simulink model "example"  (Simulink 7.0)
settings: Solver=ode4  StartTime=0.0  StopTime=100  FixedStep=0.01  RelTol=1e-3
values from neighbouring files (symbols this model uses):
  TID = min('TI' == AFT(1:2))    [PAS_callback.m]    (also in PSTID_callback.m = [block '/TID'])
libraries: simulink x280
(part 2 of 15)

== system example/<system name>/<Requirement name>/<Preconditions name>4 ==
  InOut Bus : Inport  OutDataType=sfix(16)  OutScaling=2^0
  <Reference name> : Constant  OutDataType=sfix(16)  OutScaling=2^0
  Bus Selector : BusSelector  OutputSignals=signal1
  Feature extraction : Subsystem  TreatAsAtomicUnit=on  mask{Param=0}
      mask prompts: Param "Mask Parameter 1:"
  PS : Subsystem  mask(Feature layer: preconditions synchronization){NoTI=0, NoTDD=0, NoTID=1, TIdel=[0], TDDdel=[0]}
      mask prompts: NoTI "Time-independent features identifiable with or without a delay (TI)"; NoTDD "Triggered features identifiable with determinate delay or without a delay (TDD)"; NoTID "Triggered features identifiable with indeterminate delay (TID)"; TIdel "Time-independent features delays (in time steps). E.g. [0 1 0] for 3 features"; TDDdel "Triggered features delays (in time steps). E.g. [0 0] for 2 features"
      mask help: Use this block for synchronizing the precondition features. For changing the block inputs, use the parameters below. The output must be used for assertions activation.
      mask init:
      | PS_init(gcb);
      mask StyleString: popup(0|1|2|3|4|5|6|7|8|9),popup(0|1|2|3|4|5|6|7|8|9),popup(0|1|2|3|4|5|6|7|8|9),edit,edit
      mask CallbackString:
      | PSTI_callback(gcb);|PSTDD_callback(gcb);|PSTID_callback(gcb);|NoTI = str2double(get_param(gcb,'NoTI'));
      | TIdel = str2num(get_param(gcb,'TIdel'));
      | if NoTI ~= length(TIdel) && NoTI ~= 0
      |     error(['The number of delays entered (' num2str(length(TIdel)) ') does not correspond to the above specified number of time-independent features (' num2str(NoTI) ').']);
      | end|NoTDD = str2double(get_param(gcb,'NoTDD'));
      | TDDdel = str2num(get_param(gcb,'TDDdel'));
      | if NoTDD ~= length(TDDdel) && NoTDD ~= 0
      |     error(['The number of delays entered (' num2str(length(TDDdel)) ') does not correspond to the above specified number of triggered features with constant delay (' num2str(NoTDD) ').']);
      | end
  Signal comparison : Subsystem  TreatAsAtomicUnit=on  mask{Param=0}
      mask prompts: Param "Mask Parameter 1:"
  Activate : Outport  OutDataType=sfix(16)  OutScaling=2^0
  wires:
  InOut Bus/1 -> Bus Selector/1
  PS/1(Precond) -> Activate/1
  Signal comparison/1(A) -> PS/3(A TID1)
  <Reference name>/1 -> Signal comparison/2(Ref)
  Feature extraction/3(A) -> Signal comparison/1(Sig)
  Feature extraction/2(T) -> PS/2(T TID1)
  Feature extraction/1(R) -> PS/1(R TID1)
  Bus Selector/1 -> Feature extraction/1(Sig)  "<signal1>"

== system example/<system name>/<Requirement name>/<Preconditions name>5 ==
  InOut Bus : Inport  OutDataType=sfix(16)  OutScaling=2^0
  <Reference name> : Constant  OutDataType=sfix(16)  OutScaling=2^0
  Bus Selector : BusSelector  OutputSignals=signal1
  Feature extraction : Subsystem  TreatAsAtomicUnit=on  mask{Param=0}
      mask prompts: Param "Mask Parameter 1:"
  PS : Subsystem  mask(Feature layer: preconditions synchronization){NoTI=0, NoTDD=0, NoTID=1, TIdel=[0], TDDdel=[0]}
      mask prompts: NoTI "Time-independent features identifiable with or without a delay (TI)"; NoTDD "Triggered features identifiable with determinate delay or without a delay (TDD)"; NoTID "Triggered features identifiable with indeterminate delay (TID)"; TIdel "Time-independent features delays (in time steps). E.g. [0 1 0] for 3 features"; TDDdel "Triggered features delays (in time steps). E.g. [0 0] for 2 features"
      mask help: Use this block for synchronizing the precondition features. For changing the block inputs, use the parameters below. The output must be used for assertions activation.
      mask init:
      | PS_init(gcb);
      mask StyleString: popup(0|1|2|3|4|5|6|7|8|9),popup(0|1|2|3|4|5|6|7|8|9),popup(0|1|2|3|4|5|6|7|8|9),edit,edit
      mask CallbackString:
      | PSTI_callback(gcb);|PSTDD_callback(gcb);|PSTID_callback(gcb);|NoTI = str2double(get_param(gcb,'NoTI'));
      | TIdel = str2num(get_param(gcb,'TIdel'));
      | if NoTI ~= length(TIdel) && NoTI ~= 0
      |     error(['The number of delays entered (' num2str(length(TIdel)) ') does not correspond to the above specified number of time-independent features (' num2str(NoTI) ').']);
      | end|NoTDD = str2double(get_param(gcb,'NoTDD'));
      | TDDdel = str2num(get_param(gcb,'TDDdel'));
      | if NoTDD ~= length(TDDdel) && NoTDD ~= 0
      |     error(['The number of delays entered (' num2str(length(TDDdel)) ') does not correspond to the above specified number of triggered features with constant delay (' num2str(NoTDD) ').']);
      | end
  Signal comparison : Subsystem  TreatAsAtomicUnit=on  mask{Param=0}
      mask prompts: Param "Mask Parameter 1:"
  Activate : Outport  OutDataType=sfix(16)  OutScaling=2^0
  wires:
  InOut Bus/1 -> Bus Selector/1
  PS/1(Precond) -> Activate/1
  Signal comparison/1(A) -> PS/3(A TID1)
  <Reference name>/1 -> Signal comparison/2(Ref)
  Feature extraction/3(A) -> Signal comparison/1(Sig)
  Feature extraction/2(T) -> PS/2(T TID1)
  Feature extraction/1(R) -> PS/1(R TID1)
  Bus Selector/1 -> Feature extraction/1(Sig)  "<signal1>"

== system example/<system name>/<Requirement name>/<Preconditions name>6 ==
  InOut Bus : Inport  OutDataType=sfix(16)  OutScaling=2^0
  <Reference name> : Constant  OutDataType=sfix(16)  OutScaling=2^0
  Bus Selector : BusSelector  OutputSignals=signal1
  Feature extraction : Subsystem  TreatAsAtomicUnit=on  mask{Param=0}
      mask prompts: Param "Mask Parameter 1:"
  PS : Subsystem  mask(Feature layer: preconditions synchronization){NoTI=0, NoTDD=0, NoTID=1, TIdel=[0], TDDdel=[0]}
      mask prompts: NoTI "Time-independent features identifiable with or without a delay (TI)"; NoTDD "Triggered features identifiable with determinate delay or without a delay (TDD)"; NoTID "Triggered features identifiable with indeterminate delay (TID)"; TIdel "Time-independent features delays (in time steps). E.g. [0 1 0] for 3 features"; TDDdel "Triggered features delays (in time steps). E.g. [0 0] for 2 features"
      mask help: Use this block for synchronizing the precondition features. For changing the block inputs, use the parameters below. The output must be used for assertions activation.
      mask init:
      | PS_init(gcb);
      mask StyleString: popup(0|1|2|3|4|5|6|7|8|9),popup(0|1|2|3|4|5|6|7|8|9),popup(0|1|2|3|4|5|6|7|8|9),edit,edit
      mask CallbackString:
      | PSTI_callback(gcb);|PSTDD_callback(gcb);|PSTID_callback(gcb);|NoTI = str2double(get_param(gcb,'NoTI'));
      | TIdel = str2num(get_param(gcb,'TIdel'));
      | if NoTI ~= length(TIdel) && NoTI ~= 0
      |     error(['The number of delays entered (' num2str(length(TIdel)) ') does not correspond to the above specified number of time-independent features (' num2str(NoTI) ').']);
      | end|NoTDD = str2double(get_param(gcb,'NoTDD'));
      | TDDdel = str2num(get_param(gcb,'TDDdel'));
      | if NoTDD ~= length(TDDdel) && NoTDD ~= 0
      |     error(['The number of delays entered (' num2str(length(TDDdel)) ') does not correspond to the above specified number of triggered features with constant delay (' num2str(NoTDD) ').']);
      | end
  Signal comparison : Subsystem  TreatAsAtomicUnit=on  mask{Param=0}
      mask prompts: Param "Mask Parameter 1:"
  Activate : Outport  OutDataType=sfix(16)  OutScaling=2^0
  wires:
  InOut Bus/1 -> Bus Selector/1
  PS/1(Precond) -> Activate/1
  Signal comparison/1(A) -> PS/3(A TID1)
  <Reference name>/1 -> Signal comparison/2(Ref)
  Feature extraction/3(A) -> Signal comparison/1(Sig)
  Feature extraction/2(T) -> PS/2(T TID1)
  Feature extraction/1(R) -> PS/1(R TID1)
  Bus Selector/1 -> Feature extraction/1(Sig)  "<signal1>"

== system example/<system name>/<Requirement name>2/<Assertions name> ==
  Precond : Inport  OutDataType=sfix(16)  OutScaling=2^0
  InOut Bus : Inport  Port=2  OutDataType=sfix(16)  OutScaling=2^0
  <Reference name> : Constant  OutDataType=sfix(16)  OutScaling=2^0
  Bus Creator : BusCreator  Inputs=1
  Bus Selector : BusSelector  OutputSignals=signal1
  Feature extraction : Subsystem  TreatAsAtomicUnit=on  mask{Param=0}
      mask prompts: Param "Mask Parameter 1:"
  PAS : Subsystem  mask{AFT=TID, AFD=600}
      mask prompts: AFT "Assertion feature type:"; AFD "Assertion feature delay (in time steps)"
      mask init:
      | PAS_init(gcb);
      mask StyleString: popup(TI|TDD|TID),edit
      mask CallbackString: PAS_callback(gcb);|
  Signal comparison : Subsystem  TreatAsAtomicUnit=on  mask{Param=0}
      mask prompts: Param "Mask Parameter 1:"
  VF info : Outport  OutDataType=sfix(16)  OutScaling=2^0
  wires:
  Bus Creator/1 -> VF info/1
  InOut Bus/1 -> Bus Selector/1
  Precond/1 -> PAS/1(Precond)
  PAS/1(VF Info) -> Bus Creator/1
  <Reference name>/1 -> Signal comparison/2(Ref)
  Feature extraction/3(A) -> Signal comparison/1(Sig)
  Feature extraction/2(T) -> PAS/3(T)
  Feature extraction/1(R) -> PAS/2(R)
  Bus Selector/1 -> Feature extraction/1(Sig)  "<signal1>"
  Signal comparison/1(V) -> PAS/4(V)

== system example/<system name>/<Requirement name>2/<Preconditions name> ==
  InOut Bus : Inport  OutDataType=sfix(16)  OutScaling=2^0
  <Reference name> : Constant  OutDataType=sfix(16)  OutScaling=2^0
  Bus Selector : BusSelector  OutputSignals=signal1
  Feature extraction : Subsystem  TreatAsAtomicUnit=on  mask{Param=0}
      mask prompts: Param "Mask Parameter 1:"
  PS : Subsystem  mask(Feature layer: preconditions synchronization){NoTI=0, NoTDD=0, NoTID=1, TIdel=[0], TDDdel=[0]}
      mask prompts: NoTI "Time-independent features identifiable with or without a delay (TI)"; NoTDD "Triggered features identifiable with determinate delay or without a delay (TDD)"; NoTID "Triggered features identifiable with indeterminate delay (TID)"; TIdel "Time-independent features delays (in time steps). E.g. [0 1 0] for 3 features"; TDDdel "Triggered features delays (in time steps). E.g. [0 0] for 2 features"
      mask help: Use this block for synchronizing the precondition features. For changing the block inputs, use the parameters below. The output must be used for assertions activation.
      mask init:
      | PS_init(gcb);
      mask StyleString: popup(0|1|2|3|4|5|6|7|8|9),popup(0|1|2|3|4|5|6|7|8|9),popup(0|1|2|3|4|5|6|7|8|9),edit,edit
      mask CallbackString:
      | PSTI_callback(gcb);|PSTDD_callback(gcb);|PSTID_callback(gcb);|NoTI = str2double(get_param(gcb,'NoTI'));
      | TIdel = str2num(get_param(gcb,'TIdel'));
      | if NoTI ~= length(TIdel) && NoTI ~= 0
      |     error(['The number of delays entered (' num2str(length(TIdel)) ') does not correspond to the above specified number of time-independent features (' num2str(NoTI) ').']);
      | end|NoTDD = str2double(get_param(gcb,'NoTDD'));
      | TDDdel = str2num(get_param(gcb,'TDDdel'));
      | if NoTDD ~= length(TDDdel) && NoTDD ~= 0
      |     error(['The number of delays entered (' num2str(length(TDDdel)) ') does not correspond to the above specified number of triggered features with constant delay (' num2str(NoTDD) ').']);
      | end
  Signal comparison : Subsystem  TreatAsAtomicUnit=on  mask{Param=0}
      mask prompts: Param "Mask Parameter 1:"
  Activate : Outport  OutDataType=sfix(16)  OutScaling=2^0
  wires:
  InOut Bus/1 -> Bus Selector/1
  PS/1(Precond) -> Activate/1
  Signal comparison/1(A) -> PS/3(A TID1)
  <Reference name>/1 -> Signal comparison/2(Ref)
  Feature extraction/3(A) -> Signal comparison/1(Sig)
  Feature extraction/2(T) -> PS/2(T TID1)
  Feature extraction/1(R) -> PS/1(R TID1)
  Bus Selector/1 -> Feature extraction/1(Sig)  "<signal1>"

== system example/<system name>/<Requirement name>3/<Assertions name> ==
  Precond : Inport  OutDataType=sfix(16)  OutScaling=2^0
  InOut Bus : Inport  Port=2  OutDataType=sfix(16)  OutScaling=2^0
  <Reference name> : Constant  OutDataType=sfix(16)  OutScaling=2^0
  Bus Creator : BusCreator  Inputs=1
  Bus Selector : BusSelector  OutputSignals=signal1
  Feature extraction : Subsystem  TreatAsAtomicUnit=on  mask{Param=0}
      mask prompts: Param "Mask Parameter 1:"
  PAS : Subsystem  mask{AFT=TID, AFD=600}
      mask prompts: AFT "Assertion feature type:"; AFD "Assertion feature delay (in time steps)"
      mask init:
      | PAS_init(gcb);
      mask StyleString: popup(TI|TDD|TID),edit
      mask CallbackString: PAS_callback(gcb);|
  Signal comparison : Subsystem  TreatAsAtomicUnit=on  mask{Param=0}
      mask prompts: Param "Mask Parameter 1:"
  VF info : Outport  OutDataType=sfix(16)  OutScaling=2^0
  wires:
  Bus Creator/1 -> VF info/1
  InOut Bus/1 -> Bus Selector/1
  Precond/1 -> PAS/1(Precond)
  PAS/1(VF Info) -> Bus Creator/1
  <Reference name>/1 -> Signal comparison/2(Ref)
  Feature extraction/3(A) -> Signal comparison/1(Sig)
  Feature extraction/2(T) -> PAS/3(T)
  Feature extraction/1(R) -> PAS/2(R)
  Bus Selector/1 -> Feature extraction/1(Sig)  "<signal1>"
  Signal comparison/1(V) -> PAS/4(V)

== system example/<system name>/<Requirement name>3/<Preconditions name> ==
  InOut Bus : Inport  OutDataType=sfix(16)  OutScaling=2^0
  <Reference name> : Constant  OutDataType=sfix(16)  OutScaling=2^0
  Bus Selector : BusSelector  OutputSignals=signal1
  Feature extraction : Subsystem  TreatAsAtomicUnit=on  mask{Param=0}
      mask prompts: Param "Mask Parameter 1:"
  PS : Subsystem  mask(Feature layer: preconditions synchronization){NoTI=0, NoTDD=0, NoTID=1, TIdel=[0], TDDdel=[0]}
      mask prompts: NoTI "Time-independent features identifiable with or without a delay (TI)"; NoTDD "Triggered features identifiable with determinate delay or without a delay (TDD)"; NoTID "Triggered features identifiable with indeterminate delay (TID)"; TIdel "Time-independent features delays (in time steps). E.g. [0 1 0] for 3 features"; TDDdel "Triggered features delays (in time steps). E.g. [0 0] for 2 features"
      mask help: Use this block for synchronizing the precondition features. For changing the block inputs, use the parameters below. The output must be used for assertions activation.
      mask init:
      | PS_init(gcb);
      mask StyleString: popup(0|1|2|3|4|5|6|7|8|9),popup(0|1|2|3|4|5|6|7|8|9),popup(0|1|2|3|4|5|6|7|8|9),edit,edit
      mask CallbackString:
      | PSTI_callback(gcb);|PSTDD_callback(gcb);|PSTID_callback(gcb);|NoTI = str2double(get_param(gcb,'NoTI'));
      | TIdel = str2num(get_param(gcb,'TIdel'));
      | if NoTI ~= length(TIdel) && NoTI ~= 0
      |     error(['The number of delays entered (' num2str(length(TIdel)) ') does not correspond to the above specified number of time-independent features (' num2str(NoTI) ').']);
      | end|NoTDD = str2double(get_param(gcb,'NoTDD'));
      | TDDdel = str2num(get_param(gcb,'TDDdel'));
      | if NoTDD ~= length(TDDdel) && NoTDD ~= 0
      |     error(['The number of delays entered (' num2str(length(TDDdel)) ') does not correspond to the above specified number of triggered features with constant delay (' num2str(NoTDD) ').']);
      | end
  Signal comparison : Subsystem  TreatAsAtomicUnit=on  mask{Param=0}
      mask prompts: Param "Mask Parameter 1:"
  Activate : Outport  OutDataType=sfix(16)  OutScaling=2^0
  wires:
  InOut Bus/1 -> Bus Selector/1
  PS/1(Precond) -> Activate/1
  Signal comparison/1(A) -> PS/3(A TID1)
  <Reference name>/1 -> Signal comparison/2(Ref)
  Feature extraction/3(A) -> Signal comparison/1(Sig)
  Feature extraction/2(T) -> PS/2(T TID1)
  Feature extraction/1(R) -> PS/1(R TID1)
  Bus Selector/1 -> Feature extraction/1(Sig)  "<signal1>"

== system example/<system name>/<Requirement name>4/<Assertions name> ==
  Precond : Inport  OutDataType=sfix(16)  OutScaling=2^0
  InOut Bus : Inport  Port=2  OutDataType=sfix(16)  OutScaling=2^0
  <Reference name> : Constant  OutDataType=sfix(16)  OutScaling=2^0
  Bus Creator : BusCreator  Inputs=1
  Bus Selector : BusSelector  OutputSignals=signal1
  Feature extraction : Subsystem  TreatAsAtomicUnit=on  mask{Param=0}
      mask prompts: Param "Mask Parameter 1:"
  PAS : Subsystem  mask{AFT=TID, AFD=600}
      mask prompts: AFT "Assertion feature type:"; AFD "Assertion feature delay (in time steps)"
      mask init:
      | PAS_init(gcb);
      mask StyleString: popup(TI|TDD|TID),edit
      mask CallbackString: PAS_callback(gcb);|
  Signal comparison : Subsystem  TreatAsAtomicUnit=on  mask{Param=0}
      mask prompts: Param "Mask Parameter 1:"
  VF info : Outport  OutDataType=sfix(16)  OutScaling=2^0
  wires:
  Bus Creator/1 -> VF info/1
  InOut Bus/1 -> Bus Selector/1
  Precond/1 -> PAS/1(Precond)
  PAS/1(VF Info) -> Bus Creator/1
  <Reference name>/1 -> Signal comparison/2(Ref)
  Feature extraction/3(A) -> Signal comparison/1(Sig)
  Feature extraction/2(T) -> PAS/3(T)
  Feature extraction/1(R) -> PAS/2(R)
  Bus Selector/1 -> Feature extraction/1(Sig)  "<signal1>"
  Signal comparison/1(V) -> PAS/4(V)

== system example/<system name>/<Requirement name>4/<Preconditions name> ==
  InOut Bus : Inport  OutDataType=sfix(16)  OutScaling=2^0
  <Reference name> : Constant  OutDataType=sfix(16)  OutScaling=2^0
  Bus Selector : BusSelector  OutputSignals=signal1
  Feature extraction : Subsystem  TreatAsAtomicUnit=on  mask{Param=0}
      mask prompts: Param "Mask Parameter 1:"
  PS : Subsystem  mask(Feature layer: preconditions synchronization){NoTI=0, NoTDD=0, NoTID=1, TIdel=[0], TDDdel=[0]}
      mask prompts: NoTI "Time-independent features identifiable with or without a delay (TI)"; NoTDD "Triggered features identifiable with determinate delay or without a delay (TDD)"; NoTID "Triggered features identifiable with indeterminate delay (TID)"; TIdel "Time-independent features delays (in time steps). E.g. [0 1 0] for 3 features"; TDDdel "Triggered features delays (in time steps). E.g. [0 0] for 2 features"
      mask help: Use this block for synchronizing the precondition features. For changing the block inputs, use the parameters below. The output must be used for assertions activation.
      mask init:
      | PS_init(gcb);
      mask StyleString: popup(0|1|2|3|4|5|6|7|8|9),popup(0|1|2|3|4|5|6|7|8|9),popup(0|1|2|3|4|5|6|7|8|9),edit,edit
      mask CallbackString:
      | PSTI_callback(gcb);|PSTDD_callback(gcb);|PSTID_callback(gcb);|NoTI = str2double(get_param(gcb,'NoTI'));
      | TIdel = str2num(get_param(gcb,'TIdel'));
      | if NoTI ~= length(TIdel) && NoTI ~= 0
      |     error(['The number of delays entered (' num2str(length(TIdel)) ') does not correspond to the above specified number of time-independent features (' num2str(NoTI) ').']);
      | end|NoTDD = str2double(get_param(gcb,'NoTDD'));
      | TDDdel = str2num(get_param(gcb,'TDDdel'));
      | if NoTDD ~= length(TDDdel) && NoTDD ~= 0
      |     error(['The number of delays entered (' num2str(length(TDDdel)) ') does not correspond to the above specified number of triggered features with constant delay (' num2str(NoTDD) ').']);
      | end
  Signal comparison : Subsystem  TreatAsAtomicUnit=on  mask{Param=0}
      mask prompts: Param "Mask Parameter 1:"
  Activate : Outport  OutDataType=sfix(16)  OutScaling=2^0
  wires:
  InOut Bus/1 -> Bus Selector/1
  PS/1(Precond) -> Activate/1
  Signal comparison/1(A) -> PS/3(A TID1)
  <Reference name>/1 -> Signal comparison/2(Ref)
  Feature extraction/3(A) -> Signal comparison/1(Sig)
  Feature extraction/2(T) -> PS/2(T TID1)
  Feature extraction/1(R) -> PS/1(R TID1)
  Bus Selector/1 -> Feature extraction/1(Sig)  "<signal1>"

== system example/<system name>/<Requirement name>5/<Assertions name> ==
  Precond : Inport  OutDataType=sfix(16)  OutScaling=2^0
  InOut Bus : Inport  Port=2  OutDataType=sfix(16)  OutScaling=2^0
  <Reference name> : Constant  OutDataType=sfix(16)  OutScaling=2^0
  Bus Creator : BusCreator  Inputs=1
  Bus Selector : BusSelector  OutputSignals=signal1
  Feature extraction : Subsystem  TreatAsAtomicUnit=on  mask{Param=0}
      mask prompts: Param "Mask Parameter 1:"
  PAS : Subsystem  mask{AFT=TID, AFD=600}
      mask prompts: AFT "Assertion feature type:"; AFD "Assertion feature delay (in time steps)"
      mask init:
      | PAS_init(gcb);
      mask StyleString: popup(TI|TDD|TID),edit
      mask CallbackString: PAS_callback(gcb);|
  Signal comparison : Subsystem  TreatAsAtomicUnit=on  mask{Param=0}
      mask prompts: Param "Mask Parameter 1:"
  VF info : Outport  OutDataType=sfix(16)  OutScaling=2^0
  wires:
  Bus Creator/1 -> VF info/1
  InOut Bus/1 -> Bus Selector/1
  Precond/1 -> PAS/1(Precond)
  PAS/1(VF Info) -> Bus Creator/1
  <Reference name>/1 -> Signal comparison/2(Ref)
  Feature extraction/3(A) -> Signal comparison/1(Sig)
  Feature extraction/2(T) -> PAS/3(T)
  Feature extraction/1(R) -> PAS/2(R)
  Bus Selector/1 -> Feature extraction/1(Sig)  "<signal1>"
  Signal comparison/1(V) -> PAS/4(V)

== system example/<system name>/<Requirement name>5/<Preconditions name> ==
  InOut Bus : Inport  OutDataType=sfix(16)  OutScaling=2^0
  <Reference name> : Constant  OutDataType=sfix(16)  OutScaling=2^0
  Bus Selector : BusSelector  OutputSignals=signal1
  Feature extraction : Subsystem  TreatAsAtomicUnit=on  mask{Param=0}
      mask prompts: Param "Mask Parameter 1:"
  PS : Subsystem  mask(Feature layer: preconditions synchronization){NoTI=0, NoTDD=0, NoTID=1, TIdel=[0], TDDdel=[0]}
      mask prompts: NoTI "Time-independent features identifiable with or without a delay (TI)"; NoTDD "Triggered features identifiable with determinate delay or without a delay (TDD)"; NoTID "Triggered features identifiable with indeterminate delay (TID)"; TIdel "Time-independent features delays (in time steps). E.g. [0 1 0] for 3 features"; TDDdel "Triggered features delays (in time steps). E.g. [0 0] for 2 features"
      mask help: Use this block for synchronizing the precondition features. For changing the block inputs, use the parameters below. The output must be used for assertions activation.
      mask init:
      | PS_init(gcb);
      mask StyleString: popup(0|1|2|3|4|5|6|7|8|9),popup(0|1|2|3|4|5|6|7|8|9),popup(0|1|2|3|4|5|6|7|8|9),edit,edit
      mask CallbackString:
      | PSTI_callback(gcb);|PSTDD_callback(gcb);|PSTID_callback(gcb);|NoTI = str2double(get_param(gcb,'NoTI'));
      | TIdel = str2num(get_param(gcb,'TIdel'));
      | if NoTI ~= length(TIdel) && NoTI ~= 0
      |     error(['The number of delays entered (' num2str(length(TIdel)) ') does not correspond to the above specified number of time-independent features (' num2str(NoTI) ').']);
      | end|NoTDD = str2double(get_param(gcb,'NoTDD'));
      | TDDdel = str2num(get_param(gcb,'TDDdel'));
      | if NoTDD ~= length(TDDdel) && NoTDD ~= 0
      |     error(['The number of delays entered (' num2str(length(TDDdel)) ') does not correspond to the above specified number of triggered features with constant delay (' num2str(NoTDD) ').']);
      | end
  Signal comparison : Subsystem  TreatAsAtomicUnit=on  mask{Param=0}
      mask prompts: Param "Mask Parameter 1:"
  Activate : Outport  OutDataType=sfix(16)  OutScaling=2^0
  wires:
  InOut Bus/1 -> Bus Selector/1
  PS/1(Precond) -> Activate/1
  Signal comparison/1(A) -> PS/3(A TID1)
  <Reference name>/1 -> Signal comparison/2(Ref)
  Feature extraction/3(A) -> Signal comparison/1(Sig)
  Feature extraction/2(T) -> PS/2(T TID1)
  Feature extraction/1(R) -> PS/1(R TID1)
  Bus Selector/1 -> Feature extraction/1(Sig)  "<signal1>"

== system example/<Test data generator>/<Requirement name>/<Preconditions name>/<Check> ==
  Out Bus : Inport  OutDataType=sfix(16)  OutScaling=2^0
  <Reference name> : Constant  OutDataType=sfix(16)  OutScaling=2^0
  Bus Selector : BusSelector  OutputSignals=signal1
  Memory : Memory  X0=[1]
  Signal comparison : Subsystem  TreatAsAtomicUnit=on  mask{Param=0}
      mask prompts: Param "Mask Parameter 1:"
  A : Outport  OutDataType=sfix(16)  OutScaling=2^0
  wires:
  Out Bus/1 -> Bus Selector/1
  Signal comparison/1(A) -> A/1
  Memory/1 -> Signal comparison/1(Sig)
  <Reference name>/1 -> Signal comparison/2(Ref)
  Bus Selector/1 -> Memory/1  "<SUT output>"

== system example/<Test data generator>/<Requirement name>/<Preconditions name>/Feature generation ==
  <signal1> : Outport  OutDataType=sfix(16)  OutScaling=2^0

== system example/<Test data generator>/<Requirement name>/<Preconditions name>/Feature generation2 ==
  <signal1> : Outport  OutDataType=sfix(16)  OutScaling=2^0

== system example/<Test data generator>/<Requirement name>/<Preconditions name>/Feature generation3 ==
  <signal1> : Outport  OutDataType=sfix(16)  OutScaling=2^0

== system example/<Test data generator>/<Requirement name>/<Preconditions name>/Feature generation4 ==
  <signal1> : Outport  OutDataType=sfix(16)  OutScaling=2^0

== system example/<Test data generator>/<Requirement name>/<Preconditions name>/Feature generation5 ==
  <signal1> : Outport  OutDataType=sfix(16)  OutScaling=2^0

== system example/<Test data generator>/<Requirement name>/<Preconditions name>/Feature generation6 ==
  <signal1> : Outport  OutDataType=sfix(16)  OutScaling=2^0

== system example/<Test data generator>/<Requirement name>/<Preconditions name>/Feature generation7 ==
  <signal1> : Outport  OutDataType=sfix(16)  OutScaling=2^0

== system example/<Test data generator>/<Requirement name>/Initialisation & Stabilisation/<Feature generation> ==
  <signal1> : Outport  OutDataType=sfix(16)  OutScaling=2^0

== system example/<Test data generator>/<Requirement name>2/<Preconditions name>/<Check> ==
  Out Bus : Inport  OutDataType=sfix(16)  OutScaling=2^0
  <Reference name> : Constant  OutDataType=sfix(16)  OutScaling=2^0
  Bus Selector : BusSelector  OutputSignals=signal1
  Memory : Memory  X0=[1]
  Signal comparison : Subsystem  TreatAsAtomicUnit=on  mask{Param=0}
      mask prompts: Param "Mask Parameter 1:"
  A : Outport  OutDataType=sfix(16)  OutScaling=2^0
  wires:
  Bus Selector/1 -> Memory/1  "<SUT output>"
  <Reference name>/1 -> Signal comparison/2(Ref)
  Memory/1 -> Signal comparison/1(Sig)
  Signal comparison/1(A) -> A/1
  Out Bus/1 -> Bus Selector/1

== system example/<Test data generator>/<Requirement name>2/<Preconditions name>/Feature generation ==
  <signal1> : Outport  OutDataType=sfix(16)  OutScaling=2^0

== system example/<Test data generator>/<Requirement name>2/<Preconditions name>/Feature generation2 ==
  <signal1> : Outport  OutDataType=sfix(16)  OutScaling=2^0

== system example/<Test data generator>/<Requirement name>2/<Preconditions name>/Feature generation3 ==
  <signal1> : Outport  OutDataType=sfix(16)  OutScaling=2^0

== system example/<Test data generator>/<Requirement name>2/<Preconditions name>/Feature generation4 ==
  <signal1> : Outport  OutDataType=sfix(16)  OutScaling=2^0

== system example/<Test data generator>/<Requirement name>2/<Preconditions name>/Feature generation5 ==
  <signal1> : Outport  OutDataType=sfix(16)  OutScaling=2^0

== system example/<Test data generator>/<Requirement name>2/<Preconditions name>/Feature generation6 ==
  <signal1> : Outport  OutDataType=sfix(16)  OutScaling=2^0

== system example/<Test data generator>/<Requirement name>2/<Preconditions name>/Feature generation7 ==
  <signal1> : Outport  OutDataType=sfix(16)  OutScaling=2^0

== system example/<Test data generator>/<Requirement name>2/Initialisation & Stabilisation/<Feature generation> ==
  <signal1> : Outport  OutDataType=sfix(16)  OutScaling=2^0

== system example/<Test data generator>/<Requirement name>3/<Preconditions name>/<Check> ==
  Out Bus : Inport  OutDataType=sfix(16)  OutScaling=2^0
  <Reference name> : Constant  OutDataType=sfix(16)  OutScaling=2^0
  Bus Selector : BusSelector  OutputSignals=signal1
  Memory : Memory  X0=[1]
  Signal comparison : Subsystem  TreatAsAtomicUnit=on  mask{Param=0}
      mask prompts: Param "Mask Parameter 1:"
  A : Outport  OutDataType=sfix(16)  OutScaling=2^0
  wires:
  Out Bus/1 -> Bus Selector/1
  Signal comparison/1(A) -> A/1
  Memory/1 -> Signal comparison/1(Sig)
  <Reference name>/1 -> Signal comparison/2(Ref)
  Bus Selector/1 -> Memory/1  "<SUT output>"

== system example/<Test data generator>/<Requirement name>3/<Preconditions name>/Feature generation ==
  <signal1> : Outport  OutDataType=sfix(16)  OutScaling=2^0

== system example/<Test data generator>/<Requirement name>3/<Preconditions name>/Feature generation2 ==
  <signal1> : Outport  OutDataType=sfix(16)  OutScaling=2^0

== system example/<Test data generator>/<Requirement name>3/<Preconditions name>/Feature generation3 ==
  <signal1> : Outport  OutDataType=sfix(16)  OutScaling=2^0

== system example/<Test data generator>/<Requirement name>3/<Preconditions name>/Feature generation4 ==
  <signal1> : Outport  OutDataType=sfix(16)  OutScaling=2^0

== system example/<Test data generator>/<Requirement name>3/<Preconditions name>/Feature generation5 ==
  <signal1> : Outport  OutDataType=sfix(16)  OutScaling=2^0

== system example/<Test data generator>/<Requirement name>3/<Preconditions name>/Feature generation6 ==
  <signal1> : Outport  OutDataType=sfix(16)  OutScaling=2^0

== system example/<Test data generator>/<Requirement name>3/<Preconditions name>/Feature generation7 ==
  <signal1> : Outport  OutDataType=sfix(16)  OutScaling=2^0

== system example/<Test data generator>/<Requirement name>3/Initialisation & Stabilisation/<Feature generation> ==
  <signal1> : Outport  OutDataType=sfix(16)  OutScaling=2^0

== system example/<Test data generator>/<Requirement name>4/<Preconditions name>/<Check> ==
  Out Bus : Inport  OutDataType=sfix(16)  OutScaling=2^0
  <Reference name> : Constant  OutDataType=sfix(16)  OutScaling=2^0
  Bus Selector : BusSelector  OutputSignals=signal1
  Memory : Memory  X0=[1]
  Signal comparison : Subsystem  TreatAsAtomicUnit=on  mask{Param=0}
      mask prompts: Param "Mask Parameter 1:"
  A : Outport  OutDataType=sfix(16)  OutScaling=2^0
  wires:
  Bus Selector/1 -> Memory/1  "<SUT output>"
  <Reference name>/1 -> Signal comparison/2(Ref)
  Memory/1 -> Signal comparison/1(Sig)
  Signal comparison/1(A) -> A/1
  Out Bus/1 -> Bus Selector/1

== system example/<Test data generator>/<Requirement name>4/<Preconditions name>/Feature generation ==
  <signal1> : Outport  OutDataType=sfix(16)  OutScaling=2^0

== system example/<Test data generator>/<Requirement name>4/<Preconditions name>/Feature generation2 ==
  <signal1> : Outport  OutDataType=sfix(16)  OutScaling=2^0

== system example/<Test data generator>/<Requirement name>4/<Preconditions name>/Feature generation3 ==
  <signal1> : Outport  OutDataType=sfix(16)  OutScaling=2^0

== system example/<Test data generator>/<Requirement name>4/<Preconditions name>/Feature generation4 ==
  <signal1> : Outport  OutDataType=sfix(16)  OutScaling=2^0

== system example/<Test data generator>/<Requirement name>4/<Preconditions name>/Feature generation5 ==
  <signal1> : Outport  OutDataType=sfix(16)  OutScaling=2^0

== system example/<Test data generator>/<Requirement name>4/<Preconditions name>/Feature generation6 ==
  <signal1> : Outport  OutDataType=sfix(16)  OutScaling=2^0

== system example/<Test data generator>/<Requirement name>4/<Preconditions name>/Feature generation7 ==
  <signal1> : Outport  OutDataType=sfix(16)  OutScaling=2^0

== system example/<Test data generator>/<Requirement name>4/Initialisation & Stabilisation/<Feature generation> ==
  <signal1> : Outport  OutDataType=sfix(16)  OutScaling=2^0

== system example/<system name>/<Requirement name>/<Assertions name>/Feature extraction ==
  Sig : Inport  OutDataType=sfix(16)  OutScaling=2^0
  R : Outport  OutDataType=sfix(16)  OutScaling=2^0
  T : Outport  Port=2  OutDataType=sfix(16)  OutScaling=2^0
  A : Outport  Port=3  OutDataType=sfix(16)  OutScaling=2^0
  wires:
  Sig/1 -> A/1, T/1, R/1

== system example/<system name>/<Requirement name>/<Assertions name>/PAS ==
  Precond : Inport  OutDataType=sfix(16)  OutScaling=2^0
  R : Inport  Port=2  OutDataType=sfix(16)  OutScaling=2^0
  T : Inport  Port=3  OutDataType=sfix(16)  OutScaling=2^0
  V : Inport  Port=4  OutDataType=sfix(16)  OutScaling=2^0
  A delay : Subsystem  TreatAsAtomicUnit=on  mask{Delay=600}
      mask prompts: Delay "Delay (in simulation steps) for the input signal:"
      mask init:
      | %set_param([gcb '/Discrete Transfer Fcn'],'Denominator',['[' num2str([1 zeros(1,str2double(get_param(gcb,'Delay')))]) ']']);
      mask CallbackString:
      | Delay = str2double(get_param(gcb,'Delay'));
      | if Delay < 0
      |     set_param(gcb,'Delay','0');
      |     error('Only non-negative delays are possible (causality).');
      |     set_param([gcb '/Delay'],'Value','0');
      | elseif Delay == 0
      |     set_param([gcb '/Delay'],'Value','0');
      | else
      |     set_param([gcb '/Integer Delay'],'NumDelays',num2str(Delay));
      |     set_param([gcb '/Delay'],'Value',num2str(Delay));
      | end
      mask Display: text(0.5,0.5,['z^{ ' num2str((-1)*str2double(get_param(gcb,'Delay'))) '}'],'texmode','on');
  AND1 : Logic  AllPortsSameDT=off  OutDataTypeMode=boolean
  Bus Selector : BusSelector  OutputSignals=Local verdict
  Bus Selector1 : BusSelector  OutputSignals=Expected lower limit,Expected upper limit,Actual data
  Bus Selector2 : BusSelector  OutputSignals=R,T,A
  Bus Assignment : BusAssignment  AssignedSignals=Local verdict,Delay
  Bus Assignment1 : BusAssignment  AssignedSignals=Expected lower limit,Expected upper limit,Actual data
  Constant : Constant  Value=-1  OutDataType=sfix(16)  OutScaling=2^0
  Delay bus signals : Subsystem
  Ra delay : Subsystem  TreatAsAtomicUnit=on  mask{Delay=0}
      mask prompts: Delay "Delay (in simulation steps) for the input signal:"
      mask init:
      | %set_param([gcb '/Discrete Transfer Fcn'],'Denominator',['[' num2str([1 zeros(1,str2double(get_param(gcb,'Delay')))]) ']']);
      mask CallbackString:
      | Delay = str2double(get_param(gcb,'Delay'));
      | if Delay < 0
      |     set_param(gcb,'Delay','0');
      |     error('Only non-negative delays are possible (causality).');
      |     set_param([gcb '/Delay'],'Value','0');
      | elseif Delay == 0
      |     set_param([gcb '/Delay'],'Value','0');
      | else
      |     set_param([gcb '/Integer Delay'],'NumDelays',num2str(Delay));
      |     set_param([gcb '/Delay'],'Value',num2str(Delay));
      | end
      mask Display: text(0.5,0.5,['z^{ ' num2str((-1)*str2double(get_param(gcb,'Delay'))) '}'],'texmode','on');
  Rp delay : Subsystem  TreatAsAtomicUnit=on  mask{Delay=600}
      mask prompts: Delay "Delay (in simulation steps) for the input signal:"
      mask init:
      | %set_param([gcb '/Discrete Transfer Fcn'],'Denominator',['[' num2str([1 zeros(1,str2double(get_param(gcb,'Delay')))]) ']']);
      mask CallbackString:
      | Delay = str2double(get_param(gcb,'Delay'));
      | if Delay < 0
      |     set_param(gcb,'Delay','0');
      |     error('Only non-negative delays are possible (causality).');
      |     set_param([gcb '/Delay'],'Value','0');
      | elseif Delay == 0
      |     set_param([gcb '/Delay'],'Value','0');
      | else
      |     set_param([gcb '/Integer Delay'],'NumDelays',num2str(Delay));
      |     set_param([gcb '/Delay'],'Value',num2str(Delay));
      | end
      mask Display: text(0.5,0.5,['z^{ ' num2str((-1)*str2double(get_param(gcb,'Delay'))) '}'],'texmode','on');
  Ta delay : Subsystem  TreatAsAtomicUnit=on  mask{Delay=0}
      mask prompts: Delay "Delay (in simulation steps) for the input signal:"
      mask init:
      | %set_param([gcb '/Discrete Transfer Fcn'],'Denominator',['[' num2str([1 zeros(1,str2double(get_param(gcb,'Delay')))]) ']']);
      mask CallbackString:
      | Delay = str2double(get_param(gcb,'Delay'));
      | if Delay < 0
      |     set_param(gcb,'Delay','0');
      |     error('Only non-negative delays are possible (causality).');
      |     set_param([gcb '/Delay'],'Value','0');
      | elseif Delay == 0
      |     set_param([gcb '/Delay'],'Value','0');
      | else
      |     set_param([gcb '/Integer Delay'],'NumDelays',num2str(Delay));
      |     set_param([gcb '/Delay'],'Value',num2str(Delay));
      | end
      mask Display: text(0.5,0.5,['z^{ ' num2str((-1)*str2double(get_param(gcb,'Delay'))) '}'],'texmode','on');
  Tp delay : Subsystem  TreatAsAtomicUnit=on  mask{Delay=600}
      mask prompts: Delay "Delay (in simulation steps) for the input signal:"
      mask init:
      | %set_param([gcb '/Discrete Transfer Fcn'],'Denominator',['[' num2str([1 zeros(1,str2double(get_param(gcb,'Delay')))]) ']']);
      mask CallbackString:
      | Delay = str2double(get_param(gcb,'Delay'));
      | if Delay < 0
      |     set_param(gcb,'Delay','0');
      |     error('Only non-negative delays are possible (causality).');
      |     set_param([gcb '/Delay'],'Value','0');
      | elseif Delay == 0
      |     set_param([gcb '/Delay'],'Value','0');
      | else
      |     set_param([gcb '/Integer Delay'],'NumDelays',num2str(Delay));
      |     set_param([gcb '/Delay'],'Value',num2str(Delay));
      | end
      mask Display: text(0.5,0.5,['z^{ ' num2str((-1)*str2double(get_param(gcb,'Delay'))) '}'],'texmode','on');
  V delay : Subsystem  TreatAsAtomicUnit=on  mask{Delay=0}
      mask prompts: Delay "Delay (in simulation steps) for the input signal:"
      mask init:
      | %set_param([gcb '/Discrete Transfer Fcn'],'Denominator',['[' num2str([1 zeros(1,str2double(get_param(gcb,'Delay')))]) ']']);
      mask CallbackString:
      | Delay = str2double(get_param(gcb,'Delay'));
      | if Delay < 0
      |     set_param(gcb,'Delay','0');
      |     error('Only non-negative delays are possible (causality).');
      |     set_param([gcb '/Delay'],'Value','0');
      | elseif Delay == 0
      |     set_param([gcb '/Delay'],'Value','0');
      | else
      |     set_param([gcb '/Integer Delay'],'NumDelays',num2str(Delay));
      |     set_param([gcb '/Delay'],'Value',num2str(Delay));
      | end
      mask Display: text(0.5,0.5,['z^{ ' num2str((-1)*str2double(get_param(gcb,'Delay'))) '}'],'texmode','on');
  error : Subsystem
  none - pass - fail : Subsystem
  sw D : Switch  Criteria=u2 ~= 0
  sw V : Switch  Criteria=u2 ~= 0
  VF Info : Outport  OutDataType=sfix(16)  OutScaling=2^0
  wires:
  T/1 -> Ta delay/1(In1)
  R/1 -> Ra delay/1(In1)
  V/1 -> Bus Selector/1, Bus Selector1/1, Bus Assignment1/1
  error/1(Verror) -> sw V/2, sw D/2
  Constant/1 -> sw V/1
  none - pass - fail/1(Verdict) -> sw V/3
  none - pass - fail/2(MaxDelay) -> sw D/1
  none - pass - fail/3(Delay) -> sw D/3
  sw V/1 -> Bus Assignment/2
  sw D/1 -> Bus Assignment/3
  Bus Selector/1 -> V delay/1(In1)  "<Local verdict>"
  Bus Assignment/1 -> VF Info/1
  Bus Selector2/1 -> Rp delay/1(In1)  "<R>"
  Bus Selector2/2 -> Tp delay/1(In1)  "<T>"
  Bus Selector2/3 -> A delay/1(In1)  "<A>"
  Rp delay/1(Out1) -> error/1(Rp), none - pass - fail/1(Rp), AND1/1
  Tp delay/1(Out1) -> error/2(Tp), none - pass - fail/2(Tp)
  A delay/1(Out1) -> error/3(A), none - pass - fail/3(A)
  V delay/1(Out1) -> error/6(V), none - pass - fail/6(V)
  Ra delay/1(Out1) -> none - pass - fail/4(Ra), AND1/2, error/4(Ra)
  AND1/1 -> none - pass - fail/7(R AND)
  Precond/1 -> Bus Selector2/1
  Bus Selector1/1 -> Delay bus signals/1(ELLin)  "<Expected lower limit>"
  Bus Selector1/2 -> Delay bus signals/2(EULin)  "<Expected upper limit>"
  Bus Selector1/3 -> Delay bus signals/3(ADin)  "<Actual data>"
  Bus Assignment1/1 -> Bus Assignment/1
  Delay bus signals/1(ELLout) -> Bus Assignment1/2
  Delay bus signals/2(EULout) -> Bus Assignment1/3
  Delay bus signals/3(ADout) -> Bus Assignment1/4
  Ta delay/1(Out1) -> none - pass - fail/5(Ta), error/5(Ta)

== system example/<system name>/<Requirement name>/<Assertions name>/Signal comparison ==
  Sig : Inport  OutDataType=sfix(16)  OutScaling=2^0
  Ref : Inport  Port=2  OutDataType=sfix(16)  OutScaling=2^0
  Relational Operator : RelationalOperator  Operator=<=  LogicOutDataTypeMode=boolean
  V : Outport  OutDataType=sfix(16)  OutScaling=2^0
  wires:
  Relational Operator/1 -> V/1
  Sig/1 -> Relational Operator/1
  Ref/1 -> Relational Operator/2

== system example/<system name>/<Requirement name>/<Assertions name>2/Feature extraction ==
  Sig : Inport  OutDataType=sfix(16)  OutScaling=2^0
  R : Outport  OutDataType=sfix(16)  OutScaling=2^0
  T : Outport  Port=2  OutDataType=sfix(16)  OutScaling=2^0
  A : Outport  Port=3  OutDataType=sfix(16)  OutScaling=2^0
  wires:
  Sig/1 -> A/1, T/1, R/1

== system example/<system name>/<Requirement name>/<Assertions name>2/PAS ==
  Precond : Inport  OutDataType=sfix(16)  OutScaling=2^0
  R : Inport  Port=2  OutDataType=sfix(16)  OutScaling=2^0
  T : Inport  Port=3  OutDataType=sfix(16)  OutScaling=2^0
  V : Inport  Port=4  OutDataType=sfix(16)  OutScaling=2^0
  A delay : Subsystem  TreatAsAtomicUnit=on  mask{Delay=600}
      mask prompts: Delay "Delay (in simulation steps) for the input signal:"
      mask init:
      | %set_param([gcb '/Discrete Transfer Fcn'],'Denominator',['[' num2str([1 zeros(1,str2double(get_param(gcb,'Delay')))]) ']']);
      mask CallbackString:
      | Delay = str2double(get_param(gcb,'Delay'));
      | if Delay < 0
      |     set_param(gcb,'Delay','0');
      |     error('Only non-negative delays are possible (causality).');
      |     set_param([gcb '/Delay'],'Value','0');
      | elseif Delay == 0
      |     set_param([gcb '/Delay'],'Value','0');
      | else
      |     set_param([gcb '/Integer Delay'],'NumDelays',num2str(Delay));
      |     set_param([gcb '/Delay'],'Value',num2str(Delay));
      | end
      mask Display: text(0.5,0.5,['z^{ ' num2str((-1)*str2double(get_param(gcb,'Delay'))) '}'],'texmode','on');
  AND1 : Logic  AllPortsSameDT=off  OutDataTypeMode=boolean
  Bus Selector : BusSelector  OutputSignals=Local verdict
  Bus Selector1 : BusSelector  OutputSignals=Expected lower limit,Expected upper limit,Actual data
  Bus Selector2 : BusSelector  OutputSignals=R,T,A
  Bus Assignment : BusAssignment  AssignedSignals=Local verdict,Delay
  Bus Assignment1 : BusAssignment  AssignedSignals=Expected lower limit,Expected upper limit,Actual data
  Constant : Constant  Value=-1  OutDataType=sfix(16)  OutScaling=2^0
  Delay bus signals : Subsystem
  Ra delay : Subsystem  TreatAsAtomicUnit=on  mask{Delay=0}
      mask prompts: Delay "Delay (in simulation steps) for the input signal:"
      mask init:
      | %set_param([gcb '/Discrete Transfer Fcn'],'Denominator',['[' num2str([1 zeros(1,str2double(get_param(gcb,'Delay')))]) ']']);
      mask CallbackString:
      | Delay = str2double(get_param(gcb,'Delay'));
      | if Delay < 0
      |     set_param(gcb,'Delay','0');
      |     error('Only non-negative delays are possible (causality).');
      |     set_param([gcb '/Delay'],'Value','0');
      | elseif Delay == 0
      |     set_param([gcb '/Delay'],'Value','0');
      | else
      |     set_param([gcb '/Integer Delay'],'NumDelays',num2str(Delay));
      |     set_param([gcb '/Delay'],'Value',num2str(Delay));
      | end
      mask Display: text(0.5,0.5,['z^{ ' num2str((-1)*str2double(get_param(gcb,'Delay'))) '}'],'texmode','on');
  Rp delay : Subsystem  TreatAsAtomicUnit=on  mask{Delay=600}
      mask prompts: Delay "Delay (in simulation steps) for the input signal:"
      mask init:
      | %set_param([gcb '/Discrete Transfer Fcn'],'Denominator',['[' num2str([1 zeros(1,str2double(get_param(gcb,'Delay')))]) ']']);
      mask CallbackString:
      | Delay = str2double(get_param(gcb,'Delay'));
      | if Delay < 0
      |     set_param(gcb,'Delay','0');
      |     error('Only non-negative delays are possible (causality).');
      |     set_param([gcb '/Delay'],'Value','0');
      | elseif Delay == 0
      |     set_param([gcb '/Delay'],'Value','0');
      | else
      |     set_param([gcb '/Integer Delay'],'NumDelays',num2str(Delay));
      |     set_param([gcb '/Delay'],'Value',num2str(Delay));
      | end
      mask Display: text(0.5,0.5,['z^{ ' num2str((-1)*str2double(get_param(gcb,'Delay'))) '}'],'texmode','on');
  Ta delay : Subsystem  TreatAsAtomicUnit=on  mask{Delay=0}
      mask prompts: Delay "Delay (in simulation steps) for the input signal:"
      mask init:
      | %set_param([gcb '/Discrete Transfer Fcn'],'Denominator',['[' num2str([1 zeros(1,str2double(get_param(gcb,'Delay')))]) ']']);
      mask CallbackString:
      | Delay = str2double(get_param(gcb,'Delay'));
      | if Delay < 0
      |     set_param(gcb,'Delay','0');
      |     error('Only non-negative delays are possible (causality).');
      |     set_param([gcb '/Delay'],'Value','0');
      | elseif Delay == 0
      |     set_param([gcb '/Delay'],'Value','0');
      | else
      |     set_param([gcb '/Integer Delay'],'NumDelays',num2str(Delay));
      |     set_param([gcb '/Delay'],'Value',num2str(Delay));
      | end
      mask Display: text(0.5,0.5,['z^{ ' num2str((-1)*str2double(get_param(gcb,'Delay'))) '}'],'texmode','on');
  Tp delay : Subsystem  TreatAsAtomicUnit=on  mask{Delay=600}
      mask prompts: Delay "Delay (in simulation steps) for the input signal:"
      mask init:
      | %set_param([gcb '/Discrete Transfer Fcn'],'Denominator',['[' num2str([1 zeros(1,str2double(get_param(gcb,'Delay')))]) ']']);
      mask CallbackString:
      | Delay = str2double(get_param(gcb,'Delay'));
      | if Delay < 0
      |     set_param(gcb,'Delay','0');
      |     error('Only non-negative delays are possible (causality).');
      |     set_param([gcb '/Delay'],'Value','0');
      | elseif Delay == 0
      |     set_param([gcb '/Delay'],'Value','0');
      | else
      |     set_param([gcb '/Integer Delay'],'NumDelays',num2str(Delay));
      |     set_param([gcb '/Delay'],'Value',num2str(Delay));
      | end
      mask Display: text(0.5,0.5,['z^{ ' num2str((-1)*str2double(get_param(gcb,'Delay'))) '}'],'texmode','on');
  V delay : Subsystem  TreatAsAtomicUnit=on  mask{Delay=0}
      mask prompts: Delay "Delay (in simulation steps) for the input signal:"
      mask init:
      | %set_param([gcb '/Discrete Transfer Fcn'],'Denominator',['[' num2str([1 zeros(1,str2double(get_param(gcb,'Delay')))]) ']']);
      mask CallbackString:
      | Delay = str2double(get_param(gcb,'Delay'));
      | if Delay < 0
      |     set_param(gcb,'Delay','0');
      |     error('Only non-negative delays are possible (causality).');
      |     set_param([gcb '/Delay'],'Value','0');
      | elseif Delay == 0
      |     set_param([gcb '/Delay'],'Value','0');
      | else
      |     set_param([gcb '/Integer Delay'],'NumDelays',num2str(Delay));
      |     set_param([gcb '/Delay'],'Value',num2str(Delay));
      | end
      mask Display: text(0.5,0.5,['z^{ ' num2str((-1)*str2double(get_param(gcb,'Delay'))) '}'],'texmode','on');
  error : Subsystem
  none - pass - fail : Subsystem
  sw D : Switch  Criteria=u2 ~= 0
  sw V : Switch  Criteria=u2 ~= 0
  VF Info : Outport  OutDataType=sfix(16)  OutScaling=2^0
  wires:
  T/1 -> Ta delay/1(In1)
  R/1 -> Ra delay/1(In1)
  V/1 -> Bus Selector/1, Bus Selector1/1, Bus Assignment1/1
  error/1(Verror) -> sw V/2, sw D/2
  Constant/1 -> sw V/1
  none - pass - fail/1(Verdict) -> sw V/3
  none - pass - fail/2(MaxDelay) -> sw D/1
  none - pass - fail/3(Delay) -> sw D/3
  sw V/1 -> Bus Assignment/2
  sw D/1 -> Bus Assignment/3
  Bus Selector/1 -> V delay/1(In1)  "<Local verdict>"
  Bus Assignment/1 -> VF Info/1
  Bus Selector2/1 -> Rp delay/1(In1)  "<R>"
  Bus Selector2/2 -> Tp delay/1(In1)  "<T>"
  Bus Selector2/3 -> A delay/1(In1)  "<A>"
  Rp delay/1(Out1) -> error/1(Rp), none - pass - fail/1(Rp), AND1/1
  Tp delay/1(Out1) -> error/2(Tp), none - pass - fail/2(Tp)
  A delay/1(Out1) -> error/3(A), none - pass - fail/3(A)
  V delay/1(Out1) -> error/6(V), none - pass - fail/6(V)
  Ra delay/1(Out1) -> none - pass - fail/4(Ra), AND1/2, error/4(Ra)
  AND1/1 -> none - pass - fail/7(R AND)
  Precond/1 -> Bus Selector2/1
  Bus Selector1/1 -> Delay bus signals/1(ELLin)  "<Expected lower limit>"
  Bus Selector1/2 -> Delay bus signals/2(EULin)  "<Expected upper limit>"
  Bus Selector1/3 -> Delay bus signals/3(ADin)  "<Actual data>"
  Bus Assignment1/1 -> Bus Assignment/1
  Delay bus signals/1(ELLout) -> Bus Assignment1/2
  Delay bus signals/2(EULout) -> Bus Assignment1/3
  Delay bus signals/3(ADout) -> Bus Assignment1/4
  Ta delay/1(Out1) -> none - pass - fail/5(Ta), error/5(Ta)

== system example/<system name>/<Requirement name>/<Assertions name>2/Signal comparison ==
  Sig : Inport  OutDataType=sfix(16)  OutScaling=2^0
  Ref : Inport  Port=2  OutDataType=sfix(16)  OutScaling=2^0
  Relational Operator : RelationalOperator  Operator=<=  LogicOutDataTypeMode=boolean
  V : Outport  OutDataType=sfix(16)  OutScaling=2^0
  wires:
  Relational Operator/1 -> V/1
  Sig/1 -> Relational Operator/1
  Ref/1 -> Relational Operator/2

== system example/<system name>/<Requirement name>/<Assertions name>3/Feature extraction ==
  Sig : Inport  OutDataType=sfix(16)  OutScaling=2^0
  R : Outport  OutDataType=sfix(16)  OutScaling=2^0
  T : Outport  Port=2  OutDataType=sfix(16)  OutScaling=2^0
  A : Outport  Port=3  OutDataType=sfix(16)  OutScaling=2^0
  wires:
  Sig/1 -> A/1, T/1, R/1
